simulink model "swps_2"  (Simulink 7.4)
settings: Solver=ode23s  StartTime=0.0  StopTime=inf  MaxStep=.01/50e3  RelTol=1e-3  AbsTol=1e-3
libraries: powerlib x11, simulink x8, simulink_extras x1
CloseFcn:
  | rtwprivate ssgencode ModelCloseRequest swps_2
settings Model: Creator=dbenson  LastModifiedBy=Dick
settings DataIOCC: LimitDataPoints=off  SaveOutput=off  SignalLogging=off  SaveTime=off  SignalLoggingName=sigsOut
settings OptimizationCC: BooleanDataType=off  InitFltsAndDblsToZero=on  OptimizeModelRefInitCode=on  LifeSpan=1
settings DebuggingCC: SaveWithParameterizedLinksMsg=none  SignalResolutionControl=TryResolveAllWithWarning  SolverPrmCheckMsg=none  MultiTaskDSMMsg=warning  MultiTaskCondExecSysMsg=none  StrictBusMsg=None
settings RTWCC: SystemTargetFile=ert.tlc  TemplateMakefile=ert_default_tmf  Description=Real-Time Workshop Embedded Coder (no auto configuration)  GenerateReport=on  ProcessScript=ert_make_rtw_hook  IncludeHyperlinkInReport=on  LaunchReport=on  IncludeERTFirstTime=on
settings CodeAppCC: IgnoreCustomStorageClasses=off
settings ERTTargetCC: TargetFcnLib=ansi_tfl_tmw.mat  MultiwordLength=2048  GenerateSampleERTMain=on  GenerateErtSFunction=on  InlinedParameterPlacement=NonHierarchical  ERTCustomFileTemplate=example_file_process.tlc  ConvertIfToSwitch=off

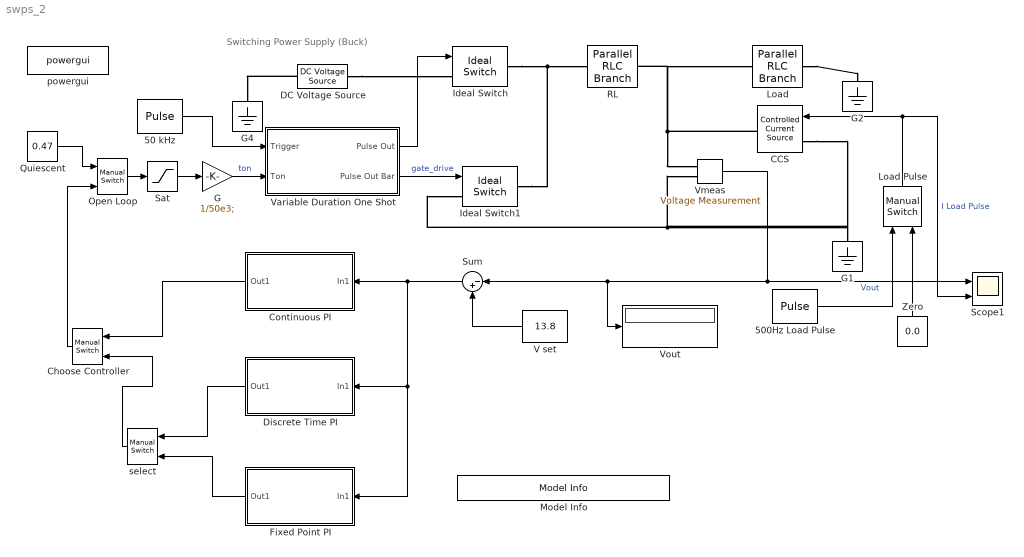
== system swps_2 ==
  note: Switching Power Supply (Buck)
  50 kHz : DiscretePulseGenerator  PulseType=Time based  Amplitude=1  Period=1/50e3;  PulseWidth=50  PhaseDelay=1e-6  SampleTime=1
  500Hz Load Pulse : DiscretePulseGenerator  PulseType=Time based  Amplitude=-2  Period=1/500  PulseWidth=50  PhaseDelay=1e-6  SampleTime=1
  CCS : powerlib/Electrical Sources/Controlled Current Source  Description=source block  DialogController=POWERSYS.PowerSysDialog  SystemSampleTime=-1  Initialize=off  Source_Type=AC  Amplitude=10  Phase=0  Frequency=0  Measurements=None
      settings: AttributesFormatString=\n
  Choose Controller : simulink/Signal Routing/Manual Switch  SystemSampleTime=-1  sw=1  action=0  varsize=off
  Continuous PI : Subsystem
  DC Voltage Source : powerlib/Electrical Sources/DC Voltage Source  Description=source block  DialogController=POWERSYS.PowerSysDialog  SystemSampleTime=-1  Amplitude=30  Measurements=None
      settings: AttributesFormatString=\n
  Discrete Time PI : Subsystem
  Fixed Point PI : Subsystem  MinMaxOverflowLogging=MinMaxAndOverflow
  G : Gain  Gain=1/50e3;  ParameterDataType=sfix(16)  ParameterScaling=2^0  OutDataType=sfix(16)  OutScaling=2^0  SaturateOnIntegerOverflow=on  OutDataTypeStr=Inherit: Same as input  ParamDataTypeStr=Inherit: Same as input
  G1 : powerlib/Elements/Ground  DialogController=POWERSYS.PowerSysDialog  PhysicalDomain=powersysdomain  SubClassName=unknown  LeftPortType=p1  RightPortType=p1  LConnTagsString=a
  G2 : powerlib/Elements/Ground  DialogController=POWERSYS.PowerSysDialog  PhysicalDomain=powersysdomain  SubClassName=unknown  LeftPortType=p1  RightPortType=p1  LConnTagsString=a
  G4 : powerlib/Elements/Ground  DialogController=POWERSYS.PowerSysDialog  PhysicalDomain=powersysdomain  SubClassName=unknown  LeftPortType=p1  RightPortType=p1  LConnTagsString=a
  Ideal Switch : powerlib/Power Electronics/Ideal Switch  DialogController=POWERSYS.PowerSysDialog  SystemSampleTime=-1  Ron=0.1  Lon=0  IC=0  Rs=0  Cs=0  Measurements=off
      settings: AttributesFormatString=\n
  Ideal Switch1 : powerlib/Power Electronics/Ideal Switch  DialogController=POWERSYS.PowerSysDialog  SystemSampleTime=-1  Ron=0.1  Lon=0  IC=0  Rs=0  Cs=0  Measurements=off
      settings: AttributesFormatString=\n
  Load : powerlib/Elements/Parallel RLC Branch  DialogController=POWERSYS.PowerSysDialog  PhysicalDomain=powersysdomain  SubClassName=unknown  LeftPortType=p1  RightPortType=p1  LConnTagsString=a  RConnTagsString=__new0  BranchType=RC  Resistance=2  Inductance=1.0  SetiL0=off  InitialCurrent=0  Capacitance=47e-6  Setx0=off  InitialVoltage=0  Measurements=None
  Load Pulse : simulink/Signal Routing/Manual Switch  SystemSampleTime=-1  sw=1  action=0  varsize=off
  Model Info : simulink/Model-Wide Utilities/Model Info  SystemSampleTime=-1  InitialBlockCM=None  BlockCM=None  Frame=on  DisplayStringWithTags=Copywrite 2005-2010 The MathWorks, Inc.  HorizontalTextAlignment=Center  LeftAlignmentValue=0.5  SourceBlockDiagram=swps_2  TagMaxNumber=20
  Open Loop : simulink/Signal Routing/Manual Switch  SystemSampleTime=-1  sw=0  action=0  varsize=off
  Quiescent : Constant  Value=0.47  OutDataType=sfix(16)  OutScaling=2^0
  RL : powerlib/Elements/Parallel RLC Branch  DialogController=POWERSYS.PowerSysDialog  PhysicalDomain=powersysdomain  SubClassName=unknown  LeftPortType=p1  RightPortType=p1  LConnTagsString=a  RConnTagsString=__new0  BranchType=RL  Resistance=10000  Inductance=1e-3  SetiL0=off  InitialCurrent=0  Capacitance=1.0  Setx0=off  InitialVoltage=0  Measurements=None
  Sat : Saturate  UpperLimit=0.95  LowerLimit=.01
  Scope1 : Scope  NumInputPorts=2
      settings: TimeRange=0.01  YMin=-5~-2.2  YMax=17.5~0.2  SaveName=ScopeData2
  Sum : Sum  Inputs=|-+  OutDataType=sfix(16)  OutScaling=2^0  SaturateOnIntegerOverflow=on  InputSameDT=on  OutDataTypeStr=Inherit: Same as first input
  "V set " : Constant  Value=13.8  OutDataType=sfix(16)  OutScaling=2^0
  Variable Duration One Shot : Subsystem
  Vmeas : powerlib/Measurements/Voltage Measurement  Tag=PoWeRsYsTeMmEaSuReMeNt  DialogController=POWERSYS.PowerSysDialog  SystemSampleTime=-1  PhasorSimulation=off  OutputType=Magnitude  PSBequivalent=0
  Vout : Display
      settings: Decimation=20
  Zero : Constant  Value=0.0  OutDataType=sfix(16)  OutScaling=2^0
  powergui : powerlib/powergui  SystemSampleTime=-1  SimulationMode=Continuous  SampleTime=0  frequency=60  SPID=off  DisableSnubberDevices=off  DisableRonSwitches=off  DisableVfSwitches=off  SwTol=0  Interpol=off  frequencyindice=0  echomessages=off  HookPort=off  DisplayEquations=off  FunctionMessages=off  EnableUseOfTLC=off  x0status=blocks  RestoreLinks=warning  Frange=[0:2:500]  Ylog=off  Xlog=on  ShowGrid=off  save=off  variable=ZData  ZoomFFT=on  StartTime=0.0  cycles=1  DisplayStyle=1  fundamental=60  FreqAxis=off  MaxFrequency=1000  frequencyindicesteady=1  RmsSteady=1  display=off  Ts=0  methode=off
  select : simulink/Signal Routing/Manual Switch  SystemSampleTime=-1  sw=1  action=0  varsize=off
  wires:
  50 kHz/1 -> Variable Duration One Shot/1(Trigger)
  "V set "/1 -> Sum/2
  Quiescent/1 -> Open Loop/1
  Open Loop/1 -> Sat/1
  G/1 -> Variable Duration One Shot/2(Ton)  "ton"
  Sat/1 -> G/1
  500Hz Load Pulse/1 -> Load Pulse/1
  Zero/1 -> Load Pulse/2
  Vmeas/1 -> Scope1/1, Sum/1, Vout/1  "Vout"
  Variable Duration One Shot/1(Pulse Out) -> Ideal Switch/1
  Variable Duration One Shot/2(Pulse Out Bar) -> Ideal Switch1/1  "gate_drive"
  Load Pulse/1 -> CCS/1, Scope1/2  "I Load Pulse"
  Choose Controller/1 -> Open Loop/2
  select/1 -> Choose Controller/2
  Continuous PI/1(Out1) -> Choose Controller/1
  Sum/1 -> Continuous PI/1(In1), Discrete Time PI/1(In1), Fixed Point PI/1(In1)
  Discrete Time PI/1(Out1) -> select/1
  Fixed Point PI/1(Out1) -> select/2
  connections:
  Load/RConn1 -- G2/LConn1
  DC Voltage Source/RConn1 -- Ideal Switch/LConn1
  RL/RConn1 -- Load/LConn1 -- Vmeas/LConn1 -- CCS/RConn1
  Ideal Switch1/RConn1 -- RL/LConn1 -- Ideal Switch/RConn1
  CCS/LConn1 -- G1/LConn1 -- Vmeas/LConn2 -- Ideal Switch1/LConn1
  DC Voltage Source/LConn1 -- G4/LConn1

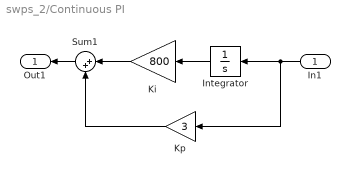
== system swps_2/Continuous PI ==
  In1 : Inport
  Integrator : Integrator
  Ki : Gain  Gain=800  ParameterDataType=sfix(16)  ParameterScaling=2^0  OutDataType=sfix(16)  OutScaling=2^0
  Kp : Gain  Gain=3  ParameterDataType=sfix(16)  ParameterScaling=2^0  OutDataType=sfix(16)  OutScaling=2^0
  Sum1 : Sum  Inputs=|++  OutDataType=sfix(16)  OutScaling=2^0  SaturateOnIntegerOverflow=on  InputSameDT=on  OutDataTypeStr=Inherit: Same as first input
  Out1 : Outport
  wires:
  In1/1 -> Kp/1, Integrator/1
  Integrator/1 -> Ki/1
  Kp/1 -> Sum1/2
  Sum1/1 -> Out1/1
  Ki/1 -> Sum1/1

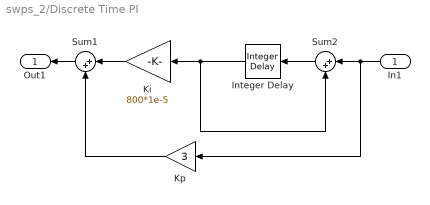
== system swps_2/Discrete Time PI ==
  In1 : Inport
  Integer Delay : simulink/Discrete/Integer Delay  vinit=0.0  samptime=1e-5  NumDelays=1
  Ki : Gain  Gain=800*1e-5  ParameterDataType=sfix(16)  ParameterScaling=2^0  OutDataType=sfix(16)  OutScaling=2^0
  Kp : Gain  Gain=3  ParameterDataType=sfix(16)  ParameterScaling=2^0  OutDataType=sfix(16)  OutScaling=2^0
  Sum1 : Sum  Inputs=|++  OutDataType=sfix(16)  OutScaling=2^0  SaturateOnIntegerOverflow=on  InputSameDT=on  OutDataTypeStr=Inherit: Same as first input
  Sum2 : Sum  Inputs=|++  OutDataType=sfix(16)  OutScaling=2^0  SaturateOnIntegerOverflow=on  InputSameDT=on  OutDataTypeStr=Inherit: Same as first input
  Out1 : Outport
  wires:
  Sum1/1 -> Out1/1
  Kp/1 -> Sum1/2
  In1/1 -> Kp/1, Sum2/1
  Integer Delay/1 -> Sum2/2, Ki/1
  Sum2/1 -> Integer Delay/1
  Ki/1 -> Sum1/1

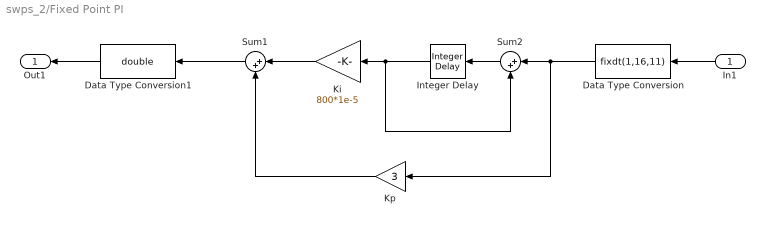
== system swps_2/Fixed Point PI ==
  In1 : Inport
  Data Type Conversion : DataTypeConversion  OutDataTypeMode=Specify via dialog  OutDataType=fixdt(1,16,11)  OutDataTypeStr=fixdt(1,16,11)  RndMeth=Nearest
  Data Type Conversion1 : DataTypeConversion  OutDataTypeMode=double  OutDataTypeStr=double  RndMeth=Nearest
  Integer Delay : simulink/Discrete/Integer Delay  vinit=0.0  samptime=1e-5  NumDelays=1
  Ki : Gain  Gain=800*1e-5  ParameterDataType=sfix(16)  ParameterScaling=2^0  OutDataTypeMode=Specify via dialog  OutDataType=fixdt(1,16,13)  OutDataTypeStr=fixdt(1,16,13)  RndMeth=Nearest
  Kp : Gain  Gain=3  ParameterDataType=sfix(16)  ParameterScaling=2^0  OutDataTypeMode=Specify via dialog  OutDataType=fixdt(1,16,9)  OutDataTypeStr=fixdt(1,16,9)  RndMeth=Nearest
  Sum1 : Sum  Inputs=|++  OutDataType=sfix(16)  OutScaling=2^0  SaturateOnIntegerOverflow=on
  Sum2 : Sum  Inputs=|++  OutDataType=sfix(16)  OutScaling=2^0  SaturateOnIntegerOverflow=on  InputSameDT=on  OutDataTypeStr=Inherit: Same as first input
  Out1 : Outport
  wires:
  Sum2/1 -> Integer Delay/1
  Integer Delay/1 -> Sum2/2, Ki/1
  In1/1 -> Data Type Conversion/1
  Kp/1 -> Sum1/2
  Sum1/1 -> Data Type Conversion1/1
  Data Type Conversion/1 -> Kp/1, Sum2/1
  Data Type Conversion1/1 -> Out1/1
  Ki/1 -> Sum1/1

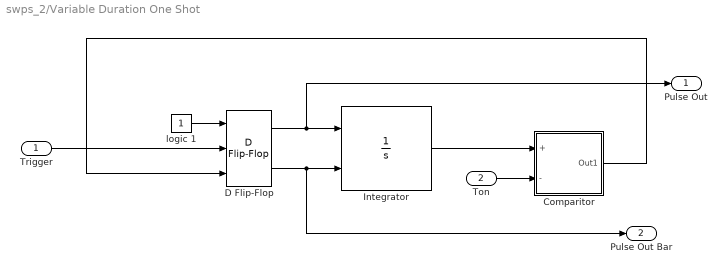
== system swps_2/Variable Duration One Shot ==
  Trigger : Inport  OutDataType=sfix(16)  OutScaling=2^0
  Ton : Inport  Port=2  OutDataType=sfix(16)  OutScaling=2^0
  Comparitor : Subsystem
  D Flip-Flop : simulink_extras/Flip Flops/D Flip-Flop  SystemSampleTime=-1
  Integrator : Integrator  ExternalReset=level
  logic 1 : Constant  OutDataType=sfix(16)  OutScaling=2^0
  Pulse Out : Outport  OutDataType=sfix(16)  OutScaling=2^0
  Pulse Out Bar : Outport  Port=2  OutDataType=sfix(16)  OutScaling=2^0
  wires:
  D Flip-Flop/2 -> Integrator/2, Pulse Out Bar/1
  logic 1/1 -> D Flip-Flop/1
  Integrator/1 -> Comparitor/1(+)
  D Flip-Flop/1 -> Integrator/1, Pulse Out/1
  Trigger/1 -> D Flip-Flop/2
  Ton/1 -> Comparitor/2(-)
  Comparitor/1(Out1) -> D Flip-Flop/3

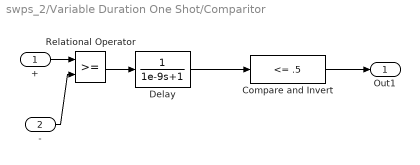
== system swps_2/Variable Duration One Shot/Comparitor ==
  + : Inport  OutDataType=sfix(16)  OutScaling=2^0
  - : Inport  Port=2  OutDataType=sfix(16)  OutScaling=2^0
  "Compare and Invert " : simulink/Logic and Bit Operations/Compare To Constant  SystemSampleTime=-1  relop=<=  const=.5  LogicOutDataTypeMode=uint8  ZeroCross=off
  Delay : TransferFcn  Denominator=[1e-9 1]
  Relational Operator : RelationalOperator  InputSameDT=on
  Out1 : Outport  OutDataType=sfix(16)  OutScaling=2^0
  wires:
  Relational Operator/1 -> Delay/1
  +/1 -> Relational Operator/1
  Delay/1 -> "Compare and Invert "/1
  -/1 -> Relational Operator/2
  "Compare and Invert "/1 -> Out1/1
